simulink model "rocketsim2"  (R2020a)
settings: Solver=VariableStepAuto  StartTime=0.0  StopTime=25  RelTol=1e-3
libraries: simulink x5, shared6dof x2, aerolibconvert2 x2, aerolibadyn x1, aerolibbdyn x1, fl_lib x1
settings Model: Creator=Rober  LastModifiedBy=Rober

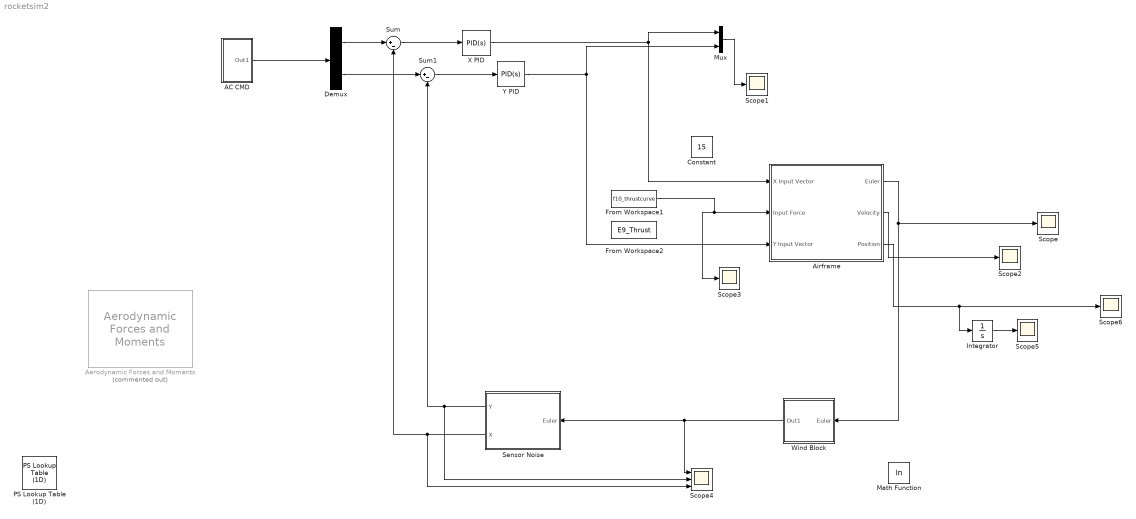
== system rocketsim2 ==
  AC CMD : Subsystem
  "Aerodynamic Forces and Moments " : aerolibadyn/Aerodynamic Forces and Moments   Commented=on  inputAxes=Body  outputForceAxes=Body  outputMomentAxes=Body  S=1  b=1  cbar=1
  Airframe : Subsystem
  Constant : Constant  Value=15
  Demux : Demux  Outputs=2
  From Workspace1 : FromWorkspace  VariableName=f10_thrustcurve
  From Workspace2 : FromWorkspace  VariableName=E9_Thrust
  Integrator : Integrator
  Math Function : Math  Operator=log  SaturateOnIntegerOverflow=on
  Mux : Mux  Inputs=2
  PS Lookup Table (1D) : fl_lib/Physical Signals/Lookup Tables/PS Lookup Table (1D)  x=[1, 2, 3, 4, 5]  f=[0, 1, 2, 3, 4]  interp_method=simscape.enum.interpolation.linear  extrap_method=simscape.enum.extrapolation.linear
      settings: SourceProductBaseCode=SS
  Scope{,1..3,5..6} (6 alike) : Scope
  Scope4 : Scope  NumInputPorts=3
  Sensor Noise : Subsystem
      settings: PortSchema="{\"entries\":[{\"content\":{\"sides\":[{\"content\":{\"connectorIds\":[\"Out1\",\"Out2\"]},\"type\":\"ConnectorPlacement.EquallySpacedRectSide\",\"uuid\":\"c60699ad-6b45-48cc-829d-b1c768687cbf\"},{\"content\":{\"connectorIds\":[\"In1\"],\"side\":\"RIGHT\"},\"type\":\"ConnectorPlacement.EquallySpacedRectSide\",\"uuid\":\"4d482381-49f8-448f-b191-db2e06747142\"},{\"content\":{\"connectorIds\":[],\"side\":\"TOP\"},\"type\":\"ConnectorPlacement.EquallySpacedRectSide\",\"uuid\":\"6a8d3cf2-ac63-490d-978b-eb33f9e74258\"}]},\"type\":\"ConnectorPlacement.EquallySpacedConnector\",\"uuid\":\"1144ef8a-7095-47b6-9bcf-12c86bfa771c\"}],\"packageUris\":[\"http://schema.mathworks.com/mf0/Connector/19700101\"],\"version\":\"1.0\"}"
  Sum : Sum  Inputs=|+-
  Sum1 : Sum  Inputs=|+-
  Wind Block : Subsystem
      settings: PortSchema="{\"entries\":[{\"content\":{\"sides\":[{\"content\":{\"connectorIds\":[\"Out1\"]},\"type\":\"ConnectorPlacement.EquallySpacedRectSide\",\"uuid\":\"076b7a5f-271f-4e29-a19f-312dd43dd9e5\"},{\"content\":{\"connectorIds\":[\"In1\"],\"side\":\"RIGHT\"},\"type\":\"ConnectorPlacement.EquallySpacedRectSide\",\"uuid\":\"e681735c-ba17-42c8-839e-e20608a1d334\"},{\"content\":{\"connectorIds\":[],\"side\":\"TOP\"},\"type\":\"ConnectorPlacement.EquallySpacedRectSide\",\"uuid\":\"c8ad3223-3c14-477c-a7e6-35567e1889fa\"}]},\"type\":\"ConnectorPlacement.EquallySpacedConnector\",\"uuid\":\"e9e5773c-1b02-479c-a706-52bdd7ac71fa\"}],\"packageUris\":[\"http://schema.mathworks.com/mf0/Connector/19700101\"],\"version\":\"1.0\"}"
  X PID : simulink/Continuous/PID Controller  Controller=PID  Form=Parallel  TimeDomain=Continuous-time  UseExternalTs=off  SampleTime=-1  IntegratorMethod=Forward Euler  FilterMethod=Forward Euler  ControllerParametersSource=internal  P=-0.0206310292526927  I=-0.000965837060148333  D=-0.108213442401603  UseFilter=on  N=5.45397025421619  TunerSelectOption=Transfer Function Based (PID Tuner App)  InitialConditionSource=internal  InitialConditionForIntegrator=0  InitialConditionForFilter=0  DifferentiatorICPrevScaledInput=0  ExternalReset=none  TrackingMode=off  Kt=1  LimitOutput=off  UpperSaturationLimit=inf  LowerSaturationLimit=-inf  LinearizeAsGain=on  AntiWindupMode=none  Kb=1  POutMin=[]  POutMax=[]  IOutMin=[]  IOutMax=[]  DOutMin=[]  DOutMax=[]  NOutMin=[]  NOutMax=[]  SumOutMin=[]  SumOutMax=[]  SaturationOutMin=[]  SaturationOutMax=[]  PParamMin=[]  PParamMax=[]  IParamMin=[]  IParamMax=[]  DParamMin=[]  DParamMax=[]  NParamMin=[]  NParamMax=[]  KbParamMin=[]  KbParamMax=[]  KtParamMin=[]  KtParamMax=[]  KbOutMin=[]  KbOutMax=[]  KtOutMin=[]  KtOutMax=[]  IntegratorOutMin=[]  IntegratorOutMax=[]  FilterOutMin=[]  FilterOutMax=[]  SumI1OutMin=[]  SumI1OutMax=[]  SumI2OutMin=[]  SumI2OutMax=[]  SumI3OutMin=[]  SumI3OutMax=[]  SumI4OutMin=[]  SumI4OutMax=[]  SumDOutMin=[]  SumDOutMax=[]  DifferentiatorOutMin=[]  DifferentiatorOutMax=[]  FilterDiffOutCoefMin=[]  FilterDiffOutCoefMax=[]  ReciprocalOutMin=[]  ReciprocalOutMax=[]  SumDenOutMin=[]  SumDenOutMax=[]  SumNumOutMin=[]  SumNumOutMax=[]  DivideOutMin=[]  DivideOutMax=[]  UdiffTsProdOutMin=[]  UdiffTsProdOutMax=[]  NTsProdOutMin=[]  NTsProdOutMax=[]  UintegralTsProdOutMin=[]  UintegralTsProdOutMax=[]  UngainTsProdOutMin=[]  UngainTsProdOutMax=[]  IntegratorContinuousStateAttributes=''  IntegratorStateMustResolveToSignalObject=off  IntegratorRTWStateStorageClass=Auto  FilterContinuousStateAttributes=''  FilterStateMustResolveToSignalObject=off  FilterRTWStateStorageClass=Auto  ParallelPVariant=InternalParameters  IdealPVariant=Disabled  IVariant=InternalParameters  DVariant=InternalParameters  IntegratorVariant=Continuous  SatVariant=Disabled  AWVariant=Passthrough  PCopyVariant=Disabled  TRVariant=Disabled  FdbkBlocksVariant=Forward  IdealPFdbkVariant=Disabled  SatFdbkVariant=Disabled  DerivativeFilterVariant=ContFilter  NVariant=InternalParameters  NCopyVariant=Disabled  FilterICVariant=InternalICsFilter  IntegratorICVariant=InternalICs  ExternalResetVariant=Disabled  TRSumVariant=Passthrough  SumFdbkVariant=Disabled  SumVariant=Sum_PID  TsampFilterVariant=InternalTs  TsampNgainVariant=Passthrough  TsampIntegralVariant=Passthrough
  Y PID : simulink/Continuous/PID Controller  Controller=PID  Form=Parallel  TimeDomain=Continuous-time  UseExternalTs=off  SampleTime=-1  IntegratorMethod=Forward Euler  FilterMethod=Forward Euler  ControllerParametersSource=internal  P=0.0206310292526927  I=0.000965837060148333  D=0.108213442401603  UseFilter=on  N=5.45397025421619  TunerSelectOption=Transfer Function Based (PID Tuner App)  InitialConditionSource=internal  InitialConditionForIntegrator=0  InitialConditionForFilter=0  DifferentiatorICPrevScaledInput=0  ExternalReset=none  TrackingMode=off  Kt=1  LimitOutput=off  UpperSaturationLimit=inf  LowerSaturationLimit=-inf  LinearizeAsGain=on  AntiWindupMode=none  Kb=1  POutMin=[]  POutMax=[]  IOutMin=[]  IOutMax=[]  DOutMin=[]  DOutMax=[]  NOutMin=[]  NOutMax=[]  SumOutMin=[]  SumOutMax=[]  SaturationOutMin=[]  SaturationOutMax=[]  PParamMin=[]  PParamMax=[]  IParamMin=[]  IParamMax=[]  DParamMin=[]  DParamMax=[]  NParamMin=[]  NParamMax=[]  KbParamMin=[]  KbParamMax=[]  KtParamMin=[]  KtParamMax=[]  KbOutMin=[]  KbOutMax=[]  KtOutMin=[]  KtOutMax=[]  IntegratorOutMin=[]  IntegratorOutMax=[]  FilterOutMin=[]  FilterOutMax=[]  SumI1OutMin=[]  SumI1OutMax=[]  SumI2OutMin=[]  SumI2OutMax=[]  SumI3OutMin=[]  SumI3OutMax=[]  SumI4OutMin=[]  SumI4OutMax=[]  SumDOutMin=[]  SumDOutMax=[]  DifferentiatorOutMin=[]  DifferentiatorOutMax=[]  FilterDiffOutCoefMin=[]  FilterDiffOutCoefMax=[]  ReciprocalOutMin=[]  ReciprocalOutMax=[]  SumDenOutMin=[]  SumDenOutMax=[]  SumNumOutMin=[]  SumNumOutMax=[]  DivideOutMin=[]  DivideOutMax=[]  UdiffTsProdOutMin=[]  UdiffTsProdOutMax=[]  NTsProdOutMin=[]  NTsProdOutMax=[]  UintegralTsProdOutMin=[]  UintegralTsProdOutMax=[]  UngainTsProdOutMin=[]  UngainTsProdOutMax=[]  IntegratorContinuousStateAttributes=''  IntegratorStateMustResolveToSignalObject=off  IntegratorRTWStateStorageClass=Auto  FilterContinuousStateAttributes=''  FilterStateMustResolveToSignalObject=off  FilterRTWStateStorageClass=Auto  ParallelPVariant=InternalParameters  IdealPVariant=Disabled  IVariant=InternalParameters  DVariant=InternalParameters  IntegratorVariant=Continuous  SatVariant=Disabled  AWVariant=Passthrough  PCopyVariant=Disabled  TRVariant=Disabled  FdbkBlocksVariant=Forward  IdealPFdbkVariant=Disabled  SatFdbkVariant=Disabled  DerivativeFilterVariant=ContFilter  NVariant=InternalParameters  NCopyVariant=Disabled  FilterICVariant=InternalICsFilter  IntegratorICVariant=InternalICs  ExternalResetVariant=Disabled  TRSumVariant=Passthrough  SumFdbkVariant=Disabled  SumVariant=Sum_PID  TsampFilterVariant=InternalTs  TsampNgainVariant=Passthrough  TsampIntegralVariant=Passthrough
  wires:
  Y PID/1 -> Mux/2, Airframe/3(Y Input Vector)
  AC CMD/1(Out1) -> Demux/1
  Demux/1 -> Sum/1
  Demux/2 -> Sum1/1
  Sum/1 -> X PID/1
  Sum1/1 -> Y PID/1
  Sensor Noise/1(Y) -> Scope4/2, Sum1/2
  Sensor Noise/2(X) -> Scope4/3, Sum/2
  X PID/1 -> Mux/1, Airframe/1(X Input Vector)
  Mux/1 -> Scope1/1
  Airframe/2(Velocity) -> Scope2/1
  Airframe/1(Euler) -> Wind Block/1(Euler), Scope/1
  Wind Block/1(Out1) -> Scope4/1, Sensor Noise/1(Euler)
  Airframe/3(Position) -> Integrator/1, Scope6/1
  Integrator/1 -> Scope5/1
  From Workspace1/1 -> Airframe/2(Input Force), Scope3/1

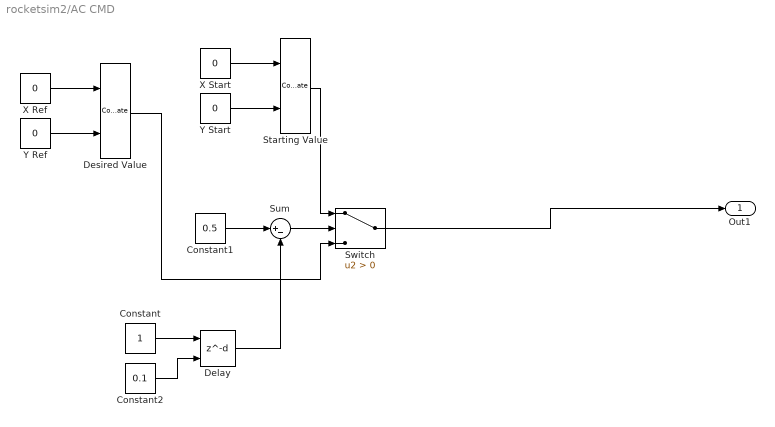
== system rocketsim2/AC CMD ==
  Constant : Constant
  Constant1 : Constant  Value=0.5
  Constant2 : Constant  Value=0.1
  Delay : Delay  DelayLengthSource=Input port  DelayLength=1  InitialCondition=0
      settings: InputPortMap=u0,p1
  Desired Value : Concatenate
  Starting Value : Concatenate
  Sum : Sum  Inputs=|+-
  Switch : Switch  Criteria=u2 > Threshold
  X Ref : Constant  Value=0
  X Start : Constant  Value=0
  Y Ref : Constant  Value=0
  Y Start : Constant  Value=0
  Out1 : Outport
  wires:
  X Ref/1 -> Desired Value/1
  Y Ref/1 -> Desired Value/2
  Desired Value/1 -> Switch/3
  Delay/1 -> Sum/2
  Constant/1 -> Delay/1
  Switch/1 -> Out1/1
  Starting Value/1 -> Switch/1
  X Start/1 -> Starting Value/1
  Y Start/1 -> Starting Value/2
  Sum/1 -> Switch/2
  Constant1/1 -> Sum/1
  Constant2/1 -> Delay/2

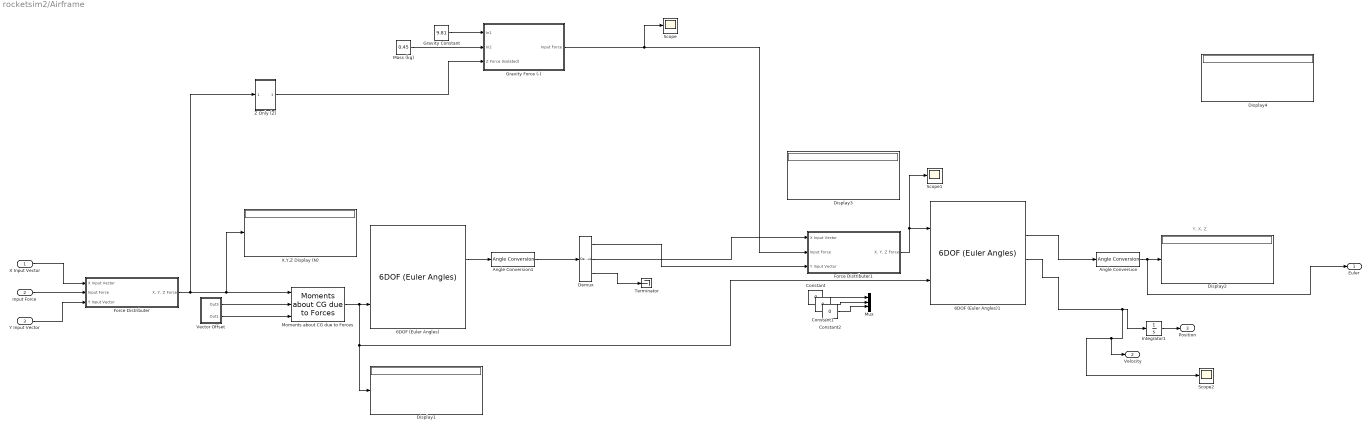
== system rocketsim2/Airframe ==
  note: Y, X, Z
  X Input Vector : Inport
  Input Force : Inport  Port=2
  Y Input Vector : Inport  Port=3
  6DOF (Euler Angles) : shared6dof/6DOF (Euler Angles)  units=Metric (MKS)  mtype=Fixed  rep=Euler Angles  xme_0=[0 0 0]  Vm_0=[0 0 0]  eul_0=[0 0 0]  pm_0=[0 0 0]  mass_0=0.45  mass_e=0.5  mass_f=2.0  inertia=eye(3)  inertia_e=eye(3)  inertia_f=2*eye(3)  k_quat=1.0  vre_flag=on  abi_flag=off  aMode=0  xme_statename=''  Vm_statename=''  eul_statename=''  quat_statename=''  pm_statename=''  mass_statename=''
      settings: SourceProductBaseCode=AE,PW,MT,VE,VP
  6DOF (Euler Angles)1 : shared6dof/6DOF (Euler Angles)  units=Metric (MKS)  mtype=Fixed  rep=Euler Angles  xme_0=[0 0 0]  Vm_0=[0 0 0]  eul_0=[0 0 0]  pm_0=[0 0 0]  mass_0=0.45  mass_e=0.5  mass_f=2.0  inertia=eye(3)  inertia_e=eye(3)  inertia_f=2*eye(3)  k_quat=1.0  vre_flag=on  abi_flag=off  aMode=0  xme_statename=''  Vm_statename=''  eul_statename=''  quat_statename=''  pm_statename=''  mass_statename=''
      settings: SourceProductBaseCode=AE,PW,MT,VE,VP
  Angle Conversion : aerolibconvert2/Angle Conversion  IU=rad  OU=deg
  Angle Conversion1 : aerolibconvert2/Angle Conversion  IU=rad  OU=deg
  Constant : Constant  Value=0
  Constant1 : Constant  Value=0
  Constant2 : Constant  Value=0
  Demux : Demux  Outputs=3
  Display{1..4} (4 alike) : Display
  Force Distributer : Subsystem
  Force Distributer1 : Subsystem
  Gravity Constant : Constant  Value=9.81
  Gravity Force (-) : Subsystem
  Integrator1 : Integrator  AbsoluteTolerance=1
  Mass (kg) : Constant  Value=0.45
  Moments about CG due to Forces : aerolibbdyn/Moments about CG  due to Forces
      settings: SourceProductBaseCode=AE
  Mux : Mux  Inputs=3
  Scope : Scope
  Scope1 : Scope
  Scope2 : Scope
  Terminator : Terminator
  Vector Offset : Subsystem
  X.Y,Z Display (N) : Display
  Z Only (Z) : Subsystem
  Euler : Outport
  Velocity : Outport  Port=2
  Position : Outport  Port=3
  wires:
  Angle Conversion/1 -> Euler/1, Display2/1
  Vector Offset/1(Out3) -> Moments about CG due to Forces/2
  Input Force/1 -> Force Distributer/2(Input Force)
  Force Distributer/1("X, Y, Z Force") -> Z Only (Z)/1(In1), Moments about CG due to Forces/1, X.Y,Z Display (N)/1
  Vector Offset/2(Out1) -> Moments about CG due to Forces/3
  Moments about CG due to Forces/1 -> 6DOF (Euler Angles)1/2, Display1/1, 6DOF (Euler Angles)/2
  X Input Vector/1 -> Force Distributer/1(X Input Vector)
  Y Input Vector/1 -> Force Distributer/3(Y Input Vector)
  Demux/3 -> Terminator/1
  Demux/2 -> Force Distributer1/1(X Input Vector)
  6DOF (Euler Angles)/3 -> Angle Conversion1/1
  Angle Conversion1/1 -> Demux/1
  Demux/1 -> Force Distributer1/3(Y Input Vector)
  Mass (kg)/1 -> Gravity Force (-)/2(In2)
  Gravity Constant/1 -> Gravity Force (-)/1(In1)
  Z Only (Z)/1(Z Force (Isolated)) -> Gravity Force (-)/3(Z Force (Isolated))
  Gravity Force (-)/1(Input Force) -> Scope/1, Force Distributer1/2(Input Force)
  Force Distributer1/1("X, Y, Z Force") -> 6DOF (Euler Angles)1/1, Scope1/1
  Integrator1/1 -> Position/1
  6DOF (Euler Angles)1/5 -> Scope2/1, Velocity/1, Integrator1/1
  6DOF (Euler Angles)1/3 -> Angle Conversion/1
  Constant2/1 -> Mux/3
  Constant1/1 -> Mux/2
  Constant/1 -> Mux/1

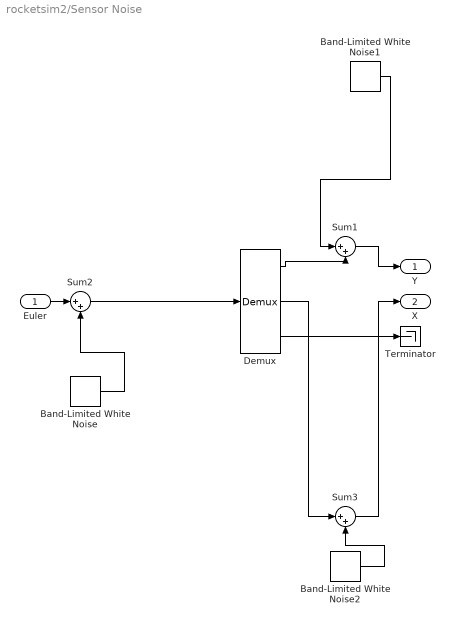
== system rocketsim2/Sensor Noise ==
  Euler : Inport
  Band-Limited White Noise : simulink/Sources/Band-Limited White Noise  Cov=[0.1]  Ts=0.1  seed=[23341]
  Band-Limited White Noise1 : simulink/Sources/Band-Limited White Noise  Cov=[0.5]  Ts=0.1  seed=[23371]
  Band-Limited White Noise2 : simulink/Sources/Band-Limited White Noise  Cov=[0.5]  Ts=0.1  seed=[23351]
  Demux : Demux  Outputs=3
  Sum1 : Sum  Inputs=|++
  Sum2 : Sum  Inputs=|++
  Sum3 : Sum  Inputs=|++
  Terminator : Terminator
  Y : Outport
  X : Outport  Port=2
  wires:
  Band-Limited White Noise/1 -> Sum2/2
  Euler/1 -> Sum2/1
  Sum2/1 -> Demux/1
  Demux/1 -> Sum1/2
  Demux/2 -> Sum3/1
  Demux/3 -> Terminator/1
  Band-Limited White Noise1/1 -> Sum1/1
  Sum1/1 -> Y/1
  Band-Limited White Noise2/1 -> Sum3/2
  Sum3/1 -> X/1

== system rocketsim2/Wind Block ==
  Euler : Inport
  Random Number : RandomNumber  Variance=80  Seed=7  SampleTime=6
  Scope7 : Scope
  Sum2 : Sum  Inputs=|++
  Out1 : Outport
  wires:
  Random Number/1 -> Scope7/1, Sum2/1
  Euler/1 -> Sum2/2
  Sum2/1 -> Out1/1

== system rocketsim2/Airframe/Force Distributer ==
  X Input Vector : Inport
  Input Force : Inport  Port=2
  Y Input Vector : Inport  Port=3
  FORCE-VECTOR CONVERSION (X,Y) : Subsystem
  FORCE-VECTOR CONVERSION (Z) : Subsystem
  "X, Y, Z Force" : Outport
  wires:
  Input Force/1 -> FORCE-VECTOR CONVERSION (Z)/2(Thrust In), FORCE-VECTOR CONVERSION (X,Y)/2(Input Force)
  FORCE-VECTOR CONVERSION (Z)/1("X, Y, Z Force") -> "X, Y, Z Force"/1
  Y Input Vector/1 -> FORCE-VECTOR CONVERSION (X,Y)/3(Y Input Vector)
  FORCE-VECTOR CONVERSION (X,Y)/1(Forces (X,Z)) -> FORCE-VECTOR CONVERSION (Z)/1("X, Y Force")
  X Input Vector/1 -> FORCE-VECTOR CONVERSION (X,Y)/1(X Input Vector)

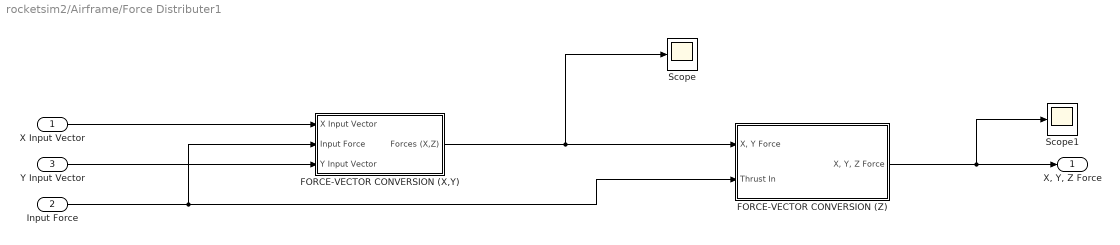
== system rocketsim2/Airframe/Force Distributer1 ==
  X Input Vector : Inport
  Input Force : Inport  Port=2
  Y Input Vector : Inport  Port=3
  FORCE-VECTOR CONVERSION (X,Y) : Subsystem
  FORCE-VECTOR CONVERSION (Z) : Subsystem
  Scope : Scope
  Scope1 : Scope
  "X, Y, Z Force" : Outport
  wires:
  Input Force/1 -> FORCE-VECTOR CONVERSION (Z)/2(Thrust In), FORCE-VECTOR CONVERSION (X,Y)/2(Input Force)
  FORCE-VECTOR CONVERSION (Z)/1("X, Y, Z Force") -> Scope1/1, "X, Y, Z Force"/1
  Y Input Vector/1 -> FORCE-VECTOR CONVERSION (X,Y)/3(Y Input Vector)
  FORCE-VECTOR CONVERSION (X,Y)/1(Forces (X,Z)) -> Scope/1, FORCE-VECTOR CONVERSION (Z)/1("X, Y Force")
  X Input Vector/1 -> FORCE-VECTOR CONVERSION (X,Y)/1(X Input Vector)

== system rocketsim2/Airframe/Gravity Force (-) ==
  In1 : Inport
  In2 : Inport  Port=2
  Z Force (Isolated) : Inport  Port=3
  Gain : Gain  Gain=-1
  Product : Product
  Scope : Scope
  Sum : Sum  Inputs=|++
  Input Force : Outport
  wires:
  Product/1 -> Gain/1
  In1/1 -> Product/1
  In2/1 -> Product/2
  Sum/1 -> Scope/1, Input Force/1
  Gain/1 -> Sum/2
  Z Force (Isolated)/1 -> Sum/1

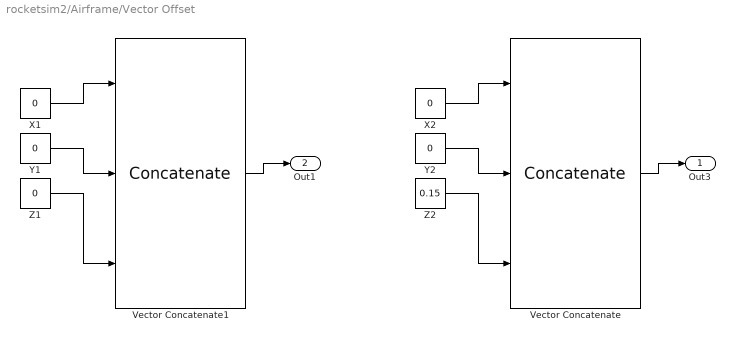
== system rocketsim2/Airframe/Vector Offset ==
  Vector Concatenate : Concatenate  NumInputs=3
  Vector Concatenate1 : Concatenate  NumInputs=3
  X1 : Constant  Value=0
  X2 : Constant  Value=0
  Y1 : Constant  Value=0
  Y2 : Constant  Value=0
  Z1 : Constant  Value=0
  Z2 : Constant  Value=0.15
  Out3 : Outport
  Out1 : Outport  Port=2
  wires:
  Z2/1 -> Vector Concatenate/3
  Y2/1 -> Vector Concatenate/2
  X2/1 -> Vector Concatenate/1
  Vector Concatenate/1 -> Out3/1
  Y1/1 -> Vector Concatenate1/2
  X1/1 -> Vector Concatenate1/1
  Vector Concatenate1/1 -> Out1/1
  Z1/1 -> Vector Concatenate1/3

== system rocketsim2/Airframe/Z Only (Z) ==
  In1 : Inport
  Demux1 : Demux  Outputs=3
  Terminator1 : Terminator
  Terminator2 : Terminator
  Z Force (Isolated) : Outport
  wires:
  Demux1/2 -> Terminator1/1
  Demux1/3 -> Z Force (Isolated)/1
  In1/1 -> Demux1/1
  Demux1/1 -> Terminator2/1

== system rocketsim2/Airframe/Force Distributer/FORCE-VECTOR CONVERSION (X,Y) ==
  X Input Vector : Inport
  Input Force : Inport  Port=2
  Y Input Vector : Inport  Port=3
  " Vector Concatenate (X,Y)" : Concatenate
  " X VECTOR FORCE CONVERSION" : Subsystem
  Display : Display
  Forces (X,Z) : Outport
  wires:
  X Input Vector/1 -> " X VECTOR FORCE CONVERSION"/1(X Vector)
  " Vector Concatenate (X,Y)"/1 -> Display/1, Forces (X,Z)/1
  Y Input Vector/1 -> " X VECTOR FORCE CONVERSION"/3(Y Vector)
  Input Force/1 -> " X VECTOR FORCE CONVERSION"/2(Input Force)
  " X VECTOR FORCE CONVERSION"/1(X) -> " Vector Concatenate (X,Y)"/1
  " X VECTOR FORCE CONVERSION"/2(Y) -> " Vector Concatenate (X,Y)"/2

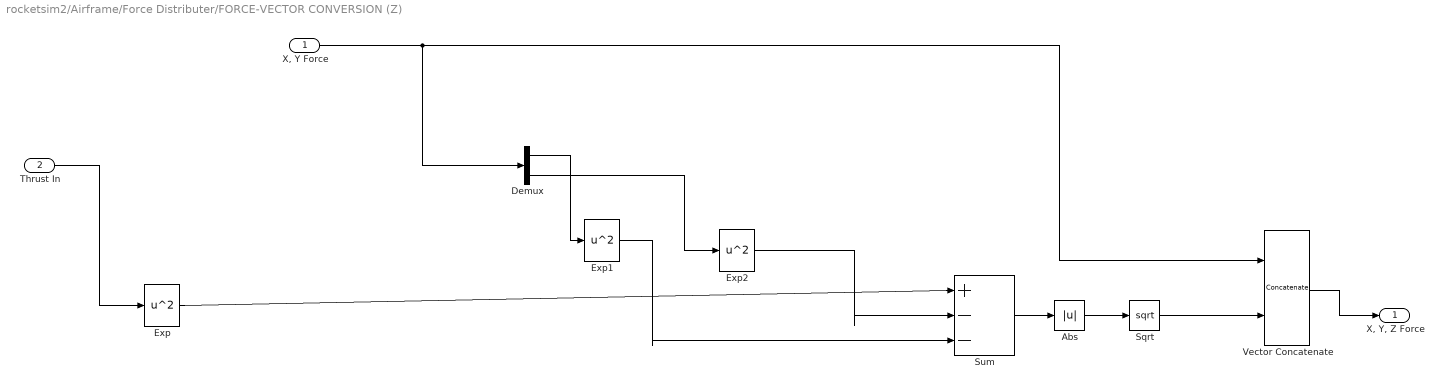
== system rocketsim2/Airframe/Force Distributer/FORCE-VECTOR CONVERSION (Z) ==
  "X, Y Force" : Inport
  Thrust In : Inport  Port=2
  Abs : Abs
  Demux : Demux  Outputs=2
  Exp : Math  Operator=square  SaturateOnIntegerOverflow=on
  Exp1 : Math  Operator=square  SaturateOnIntegerOverflow=on
  Exp2 : Math  Operator=square  SaturateOnIntegerOverflow=on
  Sqrt : Sqrt  SaturateOnIntegerOverflow=on
  Sum : Sum  Inputs=|+--
  Vector Concatenate : Concatenate
  "X, Y, Z Force" : Outport
  wires:
  "X, Y Force"/1 -> Vector Concatenate/1, Demux/1
  Abs/1 -> Sqrt/1
  Exp1/1 -> Sum/3
  Demux/1 -> Exp1/1
  Exp/1 -> Sum/1
  Demux/2 -> Exp2/1
  Thrust In/1 -> Exp/1
  Exp2/1 -> Sum/2
  Sum/1 -> Abs/1
  Sqrt/1 -> Vector Concatenate/2
  Vector Concatenate/1 -> "X, Y, Z Force"/1

== system rocketsim2/Airframe/Force Distributer1/FORCE-VECTOR CONVERSION (X,Y) ==
  X Input Vector : Inport
  Input Force : Inport  Port=2
  Y Input Vector : Inport  Port=3
  " Vector Concatenate (X,Y)" : Concatenate
  " X VECTOR FORCE CONVERSION" : Subsystem
  Display : Display
  Forces (X,Z) : Outport
  wires:
  X Input Vector/1 -> " X VECTOR FORCE CONVERSION"/1(X Vector)
  " Vector Concatenate (X,Y)"/1 -> Display/1, Forces (X,Z)/1
  Y Input Vector/1 -> " X VECTOR FORCE CONVERSION"/3(Y Vector)
  Input Force/1 -> " X VECTOR FORCE CONVERSION"/2(Input Force)
  " X VECTOR FORCE CONVERSION"/1(X) -> " Vector Concatenate (X,Y)"/1
  " X VECTOR FORCE CONVERSION"/2(Y) -> " Vector Concatenate (X,Y)"/2

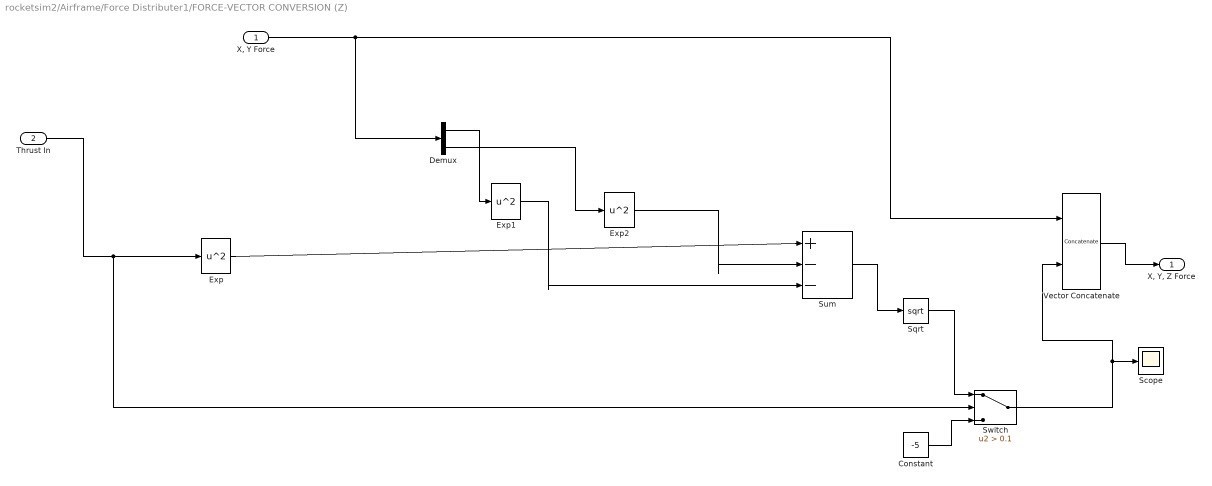
== system rocketsim2/Airframe/Force Distributer1/FORCE-VECTOR CONVERSION (Z) ==
  "X, Y Force" : Inport
  Thrust In : Inport  Port=2
  Constant : Constant  Value=-5
  Demux : Demux  Outputs=2
  Exp : Math  Operator=square  SaturateOnIntegerOverflow=on
  Exp1 : Math  Operator=square  SaturateOnIntegerOverflow=on
  Exp2 : Math  Operator=square  SaturateOnIntegerOverflow=on
  Scope : Scope
  Sqrt : Sqrt  SaturateOnIntegerOverflow=on
  Sum : Sum  Inputs=|+--
  Switch : Switch  Criteria=u2 > Threshold  Threshold=0.1
  Vector Concatenate : Concatenate
  "X, Y, Z Force" : Outport
  wires:
  "X, Y Force"/1 -> Vector Concatenate/1, Demux/1
  Exp1/1 -> Sum/3
  Demux/1 -> Exp1/1
  Exp/1 -> Sum/1
  Demux/2 -> Exp2/1
  Exp2/1 -> Sum/2
  Sqrt/1 -> Switch/1
  Vector Concatenate/1 -> "X, Y, Z Force"/1
  Thrust In/1 -> Switch/2, Exp/1
  Constant/1 -> Switch/3
  Switch/1 -> Scope/1, Vector Concatenate/2
  Sum/1 -> Sqrt/1

== system rocketsim2/Airframe/Force Distributer/FORCE-VECTOR CONVERSION (X,Y)/ X VECTOR FORCE CONVERSION ==
  X Vector : Inport
  Input Force : Inport  Port=2
  Y Vector : Inport  Port=3
  X Axis : Subsystem
  Y Axis : Subsystem
  X : Outport
  Y : Outport  Port=2
  wires:
  X Vector/1 -> X Axis/1(Input Vector)
  X Axis/1(Output X Force) -> X/1
  Y Axis/1(Output Y Force) -> Y/1
  Input Force/1 -> Y Axis/1(Input Force), X Axis/2(Input Force)
  Y Vector/1 -> Y Axis/2(Input Vector)

== system rocketsim2/Airframe/Force Distributer1/FORCE-VECTOR CONVERSION (X,Y)/ X VECTOR FORCE CONVERSION ==
  X Vector : Inport
  Input Force : Inport  Port=2
  Y Vector : Inport  Port=3
  X Axis : Subsystem
  Y Axis : Subsystem
  X : Outport
  Y : Outport  Port=2
  wires:
  X Vector/1 -> X Axis/1(Input Vector)
  X Axis/1(Output X Force) -> X/1
  Y Axis/1(Output Y Force) -> Y/1
  Input Force/1 -> Y Axis/1(Input Force), X Axis/2(Input Force)
  Y Vector/1 -> Y Axis/2(Input Vector)

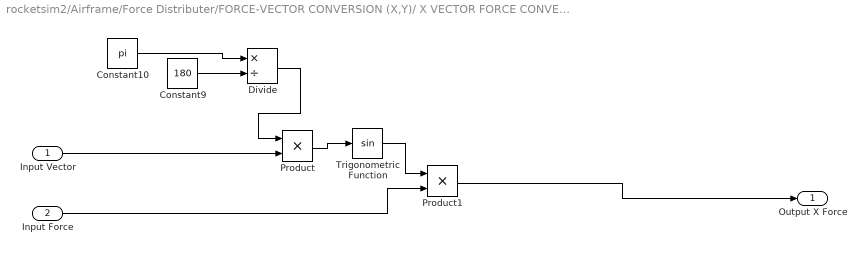
== system rocketsim2/Airframe/Force Distributer/FORCE-VECTOR CONVERSION (X,Y)/ X VECTOR FORCE CONVERSION/X Axis ==
  Input Vector : Inport
  Input Force : Inport  Port=2
  Constant10 : Constant  Value=pi
  Constant9 : Constant  Value=180
  Divide : Product  Inputs=*/
  Product : Product
  Product1 : Product
  Trigonometric Function : Trigonometry
  Output X Force : Outport
  wires:
  Product1/1 -> Output X Force/1
  Product/1 -> Trigonometric Function/1
  Input Force/1 -> Product1/2
  Input Vector/1 -> Product/2
  Constant10/1 -> Divide/1
  Trigonometric Function/1 -> Product1/1
  Constant9/1 -> Divide/2
  Divide/1 -> Product/1

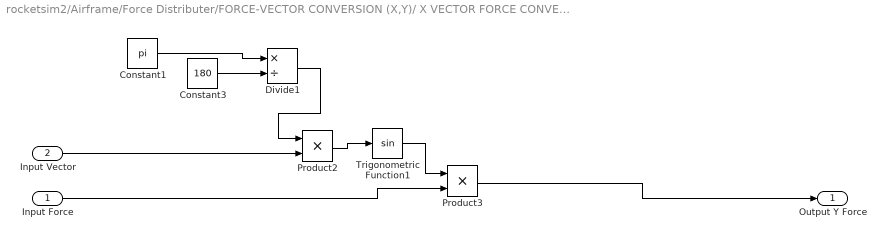
== system rocketsim2/Airframe/Force Distributer/FORCE-VECTOR CONVERSION (X,Y)/ X VECTOR FORCE CONVERSION/Y Axis ==
  Input Force : Inport
  Input Vector : Inport  Port=2
  Constant1 : Constant  Value=pi
  Constant3 : Constant  Value=180
  Divide1 : Product  Inputs=*/
  Product2 : Product
  Product3 : Product
  Trigonometric Function1 : Trigonometry
  Output Y Force : Outport
  wires:
  Product3/1 -> Output Y Force/1
  Input Vector/1 -> Product2/2
  Trigonometric Function1/1 -> Product3/1
  Constant3/1 -> Divide1/2
  Constant1/1 -> Divide1/1
  Product2/1 -> Trigonometric Function1/1
  Input Force/1 -> Product3/2
  Divide1/1 -> Product2/1

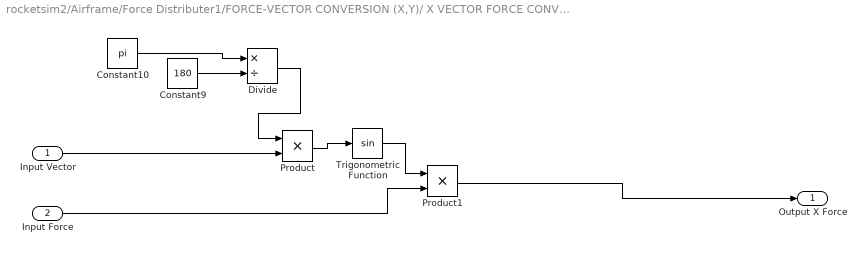
== system rocketsim2/Airframe/Force Distributer1/FORCE-VECTOR CONVERSION (X,Y)/ X VECTOR FORCE CONVERSION/X Axis ==
  Input Vector : Inport
  Input Force : Inport  Port=2
  Constant10 : Constant  Value=pi
  Constant9 : Constant  Value=180
  Divide : Product  Inputs=*/
  Product : Product
  Product1 : Product
  Trigonometric Function : Trigonometry
  Output X Force : Outport
  wires:
  Product1/1 -> Output X Force/1
  Product/1 -> Trigonometric Function/1
  Input Force/1 -> Product1/2
  Input Vector/1 -> Product/2
  Constant10/1 -> Divide/1
  Trigonometric Function/1 -> Product1/1
  Constant9/1 -> Divide/2
  Divide/1 -> Product/1

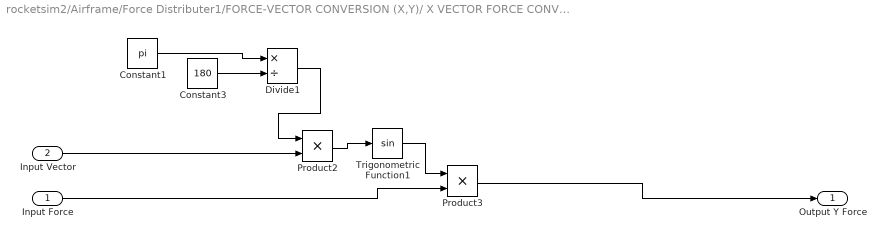
== system rocketsim2/Airframe/Force Distributer1/FORCE-VECTOR CONVERSION (X,Y)/ X VECTOR FORCE CONVERSION/Y Axis ==
  Input Force : Inport
  Input Vector : Inport  Port=2
  Constant1 : Constant  Value=pi
  Constant3 : Constant  Value=180
  Divide1 : Product  Inputs=*/
  Product2 : Product
  Product3 : Product
  Trigonometric Function1 : Trigonometry
  Output Y Force : Outport
  wires:
  Product3/1 -> Output Y Force/1
  Input Vector/1 -> Product2/2
  Trigonometric Function1/1 -> Product3/1
  Constant3/1 -> Divide1/2
  Constant1/1 -> Divide1/1
  Product2/1 -> Trigonometric Function1/1
  Input Force/1 -> Product3/2
  Divide1/1 -> Product2/1
